simulink model "Kit_Circuit"  (R2023b)
settings: Solver=VariableStepAuto  StartTime=0.0  StopTime=0.1  RelTol=1e-3
libraries: spsSeriesRLCBranchLib x11, spsGroundLib x6, spsControlledVoltageSourceLib x3, spsVoltageMeasurementLib x3, simulink x2, sps_lib x1
settings Model: Creator=Lucas  LastModifiedBy=Lucas
settings DebuggingCC: AlgebraicLoopMsg=none

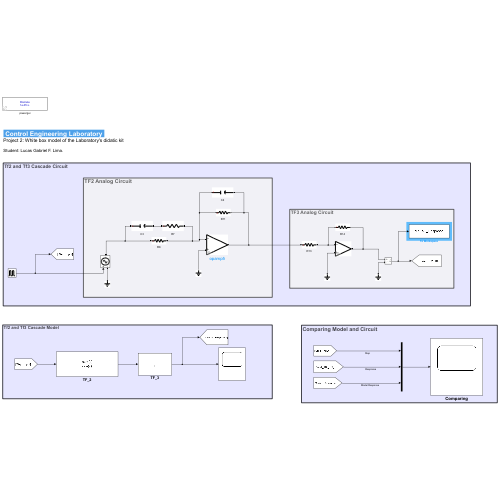
[thumbnail: Simulink's stored preview of the top-level diagram]
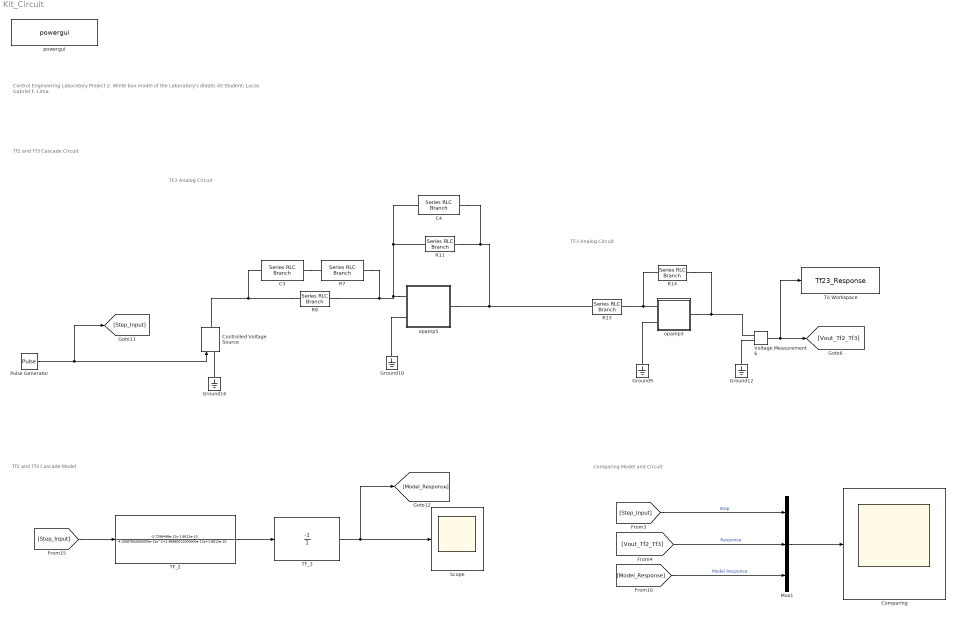
== system Kit_Circuit ==
  note: Comparing Model and Circuit
  note: Tf2 and Tf3 Cascade Model
  note: Tf2 and Tf3 Cascade Circuit
  note: TF3 Analog Circuit
  note: TF2 Analog Circuit
  note: Control Engineering Laboratory
      | Project 2: White box model of the Laboratory's didatic kit
      |
      | Student: Lucas Gabriel F. Lima.
  C3 : spsSeriesRLCBranchLib/Series RLC Branch  LConnTagsString=__new0  RConnTagsString=__new0  BranchType=C  Resistance=1  Inductance=1e-3  SetiL0=off  InitialCurrent=0  Capacitance=120e-9  Setx0=off  InitialVoltage=0  Measurements=None
  C4 : spsSeriesRLCBranchLib/Series RLC Branch  LConnTagsString=__new0  RConnTagsString=__new0  BranchType=C  Resistance=1  Inductance=1e-3  SetiL0=off  InitialCurrent=0  Capacitance=33e-9  Setx0=off  InitialVoltage=0  Measurements=None
  Comparing : Scope
  Controlled Voltage Source : spsControlledVoltageSourceLib/Controlled Voltage Source  Initialize=on  Source_Type=AC  Amplitude=0  Phase=0  Frequency=0  Measurements=None
  Ground{9..10,12,16} (4 alike) : spsGroundLib/Ground  LConnTagsString=a
  Mux1 : Mux  Inputs=3
  Pulse Generator : DiscretePulseGenerator  PulseType=Time based  Period=1/5  PulseWidth=50
  R11 : spsSeriesRLCBranchLib/Series RLC Branch  LConnTagsString=__new0  RConnTagsString=__new0  BranchType=R  Resistance=47e3  Inductance=1e-3  SetiL0=off  InitialCurrent=0  Capacitance=1e-6  Setx0=off  InitialVoltage=0  Measurements=None
  R13 : spsSeriesRLCBranchLib/Series RLC Branch  LConnTagsString=__new0  RConnTagsString=__new0  BranchType=R  Resistance=1e6  Inductance=1e-3  SetiL0=off  InitialCurrent=0  Capacitance=1e-6  Setx0=off  InitialVoltage=0  Measurements=None
  R14 : spsSeriesRLCBranchLib/Series RLC Branch  LConnTagsString=__new0  RConnTagsString=__new0  BranchType=R  Resistance=1e6  Inductance=1e-3  SetiL0=off  InitialCurrent=0  Capacitance=1e-6  Setx0=off  InitialVoltage=0  Measurements=None
  R7 : spsSeriesRLCBranchLib/Series RLC Branch  LConnTagsString=__new0  RConnTagsString=__new0  BranchType=R  Resistance=120e3  Inductance=1e-3  SetiL0=off  InitialCurrent=0  Capacitance=1e-6  Setx0=off  InitialVoltage=0  Measurements=None
  R8 : spsSeriesRLCBranchLib/Series RLC Branch  LConnTagsString=__new0  RConnTagsString=__new0  BranchType=R  Resistance=47e3  Inductance=1e-3  SetiL0=off  InitialCurrent=0  Capacitance=1e-6  Setx0=off  InitialVoltage=0  Measurements=None
  Scope : Scope
  TF_2 : TransferFcn  Numerator=[-3.7298448e-12 -1.8612e-10]  Denominator=[4.15687852800000e-15 2.96880012000000e-12 1.8612e-10]
  TF_3 : TransferFcn  Numerator=[-1]  Denominator=[1]
  To Workspace : ToWorkspace  VariableName=Tf23_Response  SaveFormat=Structure With Time  SampleTime=-1
  Voltage Measurement6 : spsVoltageMeasurementLib/Voltage Measurement  PhasorSimulation=off  OutputType=Complex  PSBequivalent=0
  opamp3 : Subsystem  mask(Opamp){Ri=1e7, Ro=100, A=200000, U1=12, U2=-12}
      mask prompts: Ri "Input Resistance"; Ro "Output Resistance"; A "Open loop amplification"; U1 "Upper limit supply voltage"; U2 "Lower limit supply voltage"
      mask Display:
      | plot([10 20 30 40], [10 12 14 16],[10 20 30 40], [22 20 18 16],[10 10],[10 22])
      | text(10,13.4,'+')
      | text(10,21,'_')
  opamp5 : Subsystem  mask(Opamp){Ri=1e7, Ro=100, A=200000, U1=12, U2=-12}
      mask prompts: Ri "Input Resistance"; Ro "Output Resistance"; A "Open loop amplification"; U1 "Upper limit supply voltage"; U2 "Lower limit supply voltage"
      mask Display:
      | plot([10 20 30 40], [10 12 14 16],[10 20 30 40], [22 20 18 16],[10 10],[10 22])
      | text(10,13.4,'+')
      | text(10,21,'_')
  powergui : sps_lib/powergui  Priority=1  SimulationMode=Discrete  SampleTime=1e-5  frequency=60  Iterations=50  frequencyindice=0  Pbase=100e6  ErrMax=1e-4  UnitsV=kV  UnitsW=MW  buscounter=0  FunctionMessages=off  echomessages=off  EnableUseOfTLC=off  CurrentSourceSwitches=off  DisableSnubberDevices=off  DisableRonSwitches=off  DisableVfSwitches=off  DisplayEquations=off  AutomaticDiscreteSolvers=off  SolverType=Tustin/Backward Euler (TBE)  Interpol=off  ExternalGateDelay=off  methode=off  Ts=100  x0status=blocks  SPID=off  SwTol=0  HookPort=off  NonlinearTolerance=1e-4  nMaxIteration=100  ContinueOnMaxIteration=off  RestoreLinks=warning  ResistiveCurrentMeasurement=off  Frange=[0:2:500]  Ylog=off  Xlog=on  ShowGrid=off  save=off  variable=ZData  structure=0  ZoomFFT=off  StartTime=0.0  cycles=1  DisplayStyle=1  fundamental=60  FreqAxis=off  MaxFrequency=1000  frequencyindicesteady=1  RmsSteady=1  display=off
  wires:
  Voltage Measurement6/1 -> [Vout_Tf2_Tf3], To Workspace/1
  Pulse Generator/1 -> [Step_Input], Controlled Voltage Source/1
  Mux1/1 -> Comparing/1
  [Step_Input] -> TF_2/1
  TF_2/1 -> TF_3/1
  TF_3/1 -> Scope/1, [Model_Response]
  [Step_Input] -> Mux1/1  "Step"
  [Model_Response] -> Mux1/3  "Model Response"
  [Vout_Tf2_Tf3] -> Mux1/2  "Response"
  connections:
  R14/RConn1 -- Voltage Measurement6/LConn1 -- opamp3/RConn1
  opamp5/RConn1 -- C4/RConn1 -- R11/RConn1 -- R13/LConn1
  R14/LConn1 -- R13/RConn1 -- opamp3/LConn1
  Ground12/LConn1 -- Voltage Measurement6/LConn2
  Ground9/LConn1 -- opamp3/LConn2
  R8/LConn1 -- C3/LConn1 -- Controlled Voltage Source/RConn1
  opamp5/LConn1 -- C4/LConn1 -- R11/LConn1 -- R7/RConn1 -- R8/RConn1
  Ground16/LConn1 -- Controlled Voltage Source/LConn1
  Ground10/LConn1 -- opamp5/LConn2
  C3/RConn1 -- R7/LConn1

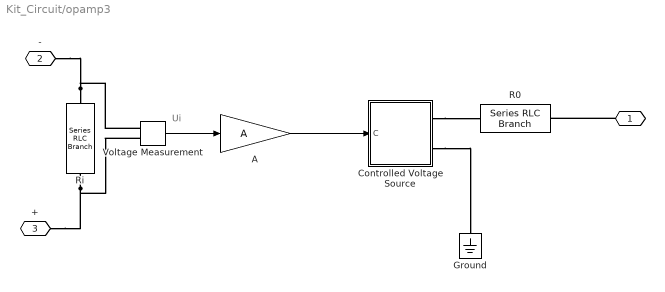
== system Kit_Circuit/opamp3 ==
  note: Ui
  A : Gain  Gain=A
  Controlled Voltage Source : Subsystem
  Ground : spsGroundLib/Ground  LConnTagsString=a
  R0 : spsSeriesRLCBranchLib/Series RLC Branch  LConnTagsString=__new0  RConnTagsString=__new0  BranchType=R  Resistance=Ro  Inductance=1.0  SetiL0=off  InitialCurrent=0  Capacitance=1.0  Setx0=off  InitialVoltage=0  Measurements=None
  Ri : spsSeriesRLCBranchLib/Series RLC Branch  LConnTagsString=__new0  RConnTagsString=__new0  BranchType=R  Resistance=Ri  Inductance=1.0  SetiL0=off  InitialCurrent=0  Capacitance=1.0  Setx0=off  InitialVoltage=0  Measurements=None
  Voltage Measurement : spsVoltageMeasurementLib/Voltage Measurement  PhasorSimulation=off  OutputType=Complex  PSBequivalent=0
  " " : PMIOPort  Side=Right
  - : PMIOPort  Port=2  Side=Left
  + : PMIOPort  Port=3  Side=Left
  wires:
  A/1 -> Controlled Voltage Source/1(C)
  Voltage Measurement/1 -> A/1
  connections:
  Controlled Voltage Source/RConn2 -- Ground/LConn1
  Ri/RConn1 -- Voltage Measurement/LConn2 -- +/RConn1
  Ri/LConn1 -- Voltage Measurement/LConn1 -- -/RConn1
  Controlled Voltage Source/RConn1 -- R0/RConn1
  " "/RConn1 -- R0/LConn1

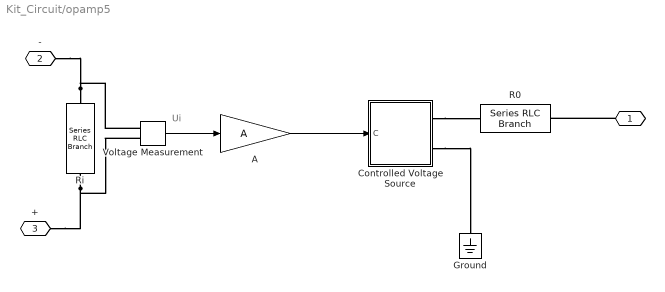
== system Kit_Circuit/opamp5 ==
  note: Ui
  A : Gain  Gain=A
  Controlled Voltage Source : Subsystem
  Ground : spsGroundLib/Ground  LConnTagsString=a
  R0 : spsSeriesRLCBranchLib/Series RLC Branch  LConnTagsString=__new0  RConnTagsString=__new0  BranchType=R  Resistance=Ro  Inductance=1.0  SetiL0=off  InitialCurrent=0  Capacitance=1.0  Setx0=off  InitialVoltage=0  Measurements=None
  Ri : spsSeriesRLCBranchLib/Series RLC Branch  LConnTagsString=__new0  RConnTagsString=__new0  BranchType=R  Resistance=Ri  Inductance=1.0  SetiL0=off  InitialCurrent=0  Capacitance=1.0  Setx0=off  InitialVoltage=0  Measurements=None
  Voltage Measurement : spsVoltageMeasurementLib/Voltage Measurement  PhasorSimulation=off  OutputType=Complex  PSBequivalent=0
  " " : PMIOPort  Side=Right
  - : PMIOPort  Port=2  Side=Left
  + : PMIOPort  Port=3  Side=Left
  wires:
  A/1 -> Controlled Voltage Source/1(C)
  Voltage Measurement/1 -> A/1
  connections:
  Controlled Voltage Source/RConn2 -- Ground/LConn1
  Ri/RConn1 -- Voltage Measurement/LConn2 -- +/RConn1
  Ri/LConn1 -- Voltage Measurement/LConn1 -- -/RConn1
  Controlled Voltage Source/RConn1 -- R0/RConn1
  " "/RConn1 -- R0/LConn1

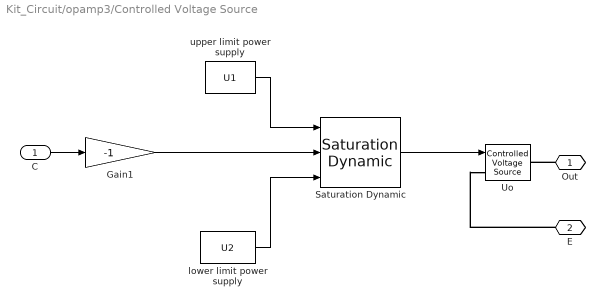
== system Kit_Circuit/opamp3/Controlled Voltage Source ==
  C : Inport
  Gain1 : Gain  Gain=-1
  Saturation Dynamic : simulink/Discontinuities/Saturation Dynamic  OutMin=[]  OutMax=[]  OutDataTypeStr=Inherit: Same as second input  OutDataType=fixdt(1, 16)  OutScaling=2^-10  DoSatur=off
  Uo : spsControlledVoltageSourceLib/Controlled Voltage Source  Initialize=off  Source_Type=AC  Amplitude=0  Phase=0  Frequency=0  Measurements=None
  lower limit power supply : Constant  Value=U2
  upper limit power supply : Constant  Value=U1
  Out : PMIOPort  Side=Right
  E : PMIOPort  Port=2  Side=Right
  wires:
  Gain1/1 -> Saturation Dynamic/2
  lower limit power supply/1 -> Saturation Dynamic/3
  upper limit power supply/1 -> Saturation Dynamic/1
  C/1 -> Gain1/1
  Saturation Dynamic/1 -> Uo/1
  connections:
  Out/RConn1 -- Uo/RConn1
  E/RConn1 -- Uo/LConn1

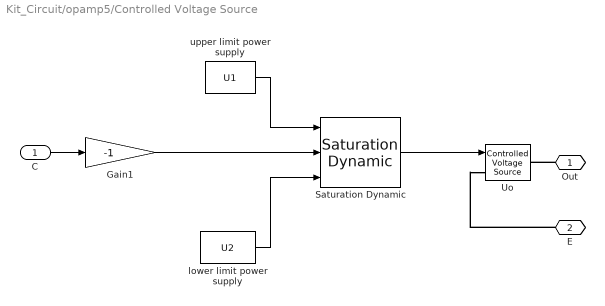
== system Kit_Circuit/opamp5/Controlled Voltage Source ==
  C : Inport
  Gain1 : Gain  Gain=-1
  Saturation Dynamic : simulink/Discontinuities/Saturation Dynamic  OutMin=[]  OutMax=[]  OutDataTypeStr=Inherit: Same as second input  OutDataType=fixdt(1, 16)  OutScaling=2^-10  DoSatur=off
  Uo : spsControlledVoltageSourceLib/Controlled Voltage Source  Initialize=off  Source_Type=AC  Amplitude=0  Phase=0  Frequency=0  Measurements=None
  lower limit power supply : Constant  Value=U2
  upper limit power supply : Constant  Value=U1
  Out : PMIOPort  Side=Right
  E : PMIOPort  Port=2  Side=Right
  wires:
  Gain1/1 -> Saturation Dynamic/2
  lower limit power supply/1 -> Saturation Dynamic/3
  upper limit power supply/1 -> Saturation Dynamic/1
  C/1 -> Gain1/1
  Saturation Dynamic/1 -> Uo/1
  connections:
  Out/RConn1 -- Uo/RConn1
  E/RConn1 -- Uo/LConn1
